simulink model "Flanging"  (R2018b)
settings: Solver=VariableStepAuto  StartTime=0.0  StopTime=10.0  RelTol=1e-3
libraries: dspsnks4 x1, dspvision x1
settings Model: Creator=alexa  LastModifiedBy=alexa

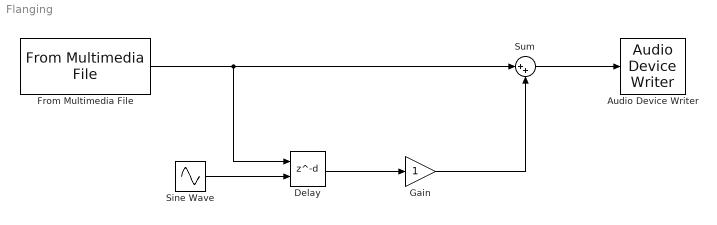
== system Flanging ==
  Audio Device Writer : dspsnks4/Audio Device Writer  Driver=DirectSound  Device=Default  InheritSampleRate=on  SampleRate=44100  BitDepth=16-bit integer  BufferSize=4096  NumBuffers=10  DefaultOutputChannelMapping=on  OutputChannelMapping=1:2  OutputNumUnderrunSamples=off  DriverIdx=1  DeviceWarnFlag=''
  Delay : Delay  DelayLengthSource=Input port
      settings: InputPortMap=u0,p1
  From Multimedia File : dspvision/From Multimedia File  inputFilename=C:\Users\alexa\OneDrive\Documents\Codigos PDS\Clase 3\Sonido.wav  loop=on  numPlays=inf  outputStreams=Audio only  videoDataType=single  audioDataType=double  inheritSampleTime=on  userDefinedSampleTime=1/30  noAudioOutput=off  isIntensityVideo=off  fourcc=RGB  colorVideoFormat=Separate color signals  outputEOF=off  dataOrg=Column-major  audioFrameSize=1024  computeAudioFrameSize=off  outSamplingMode=Sample based
      settings: SourceProductBaseCode=VP
  Gain : Gain
  Sine Wave : Sin  Amplitude=10  SampleTime=0
  Sum : Sum  Inputs=|++
  wires:
  From Multimedia File/1 -> Delay/1, Sum/1
  Sum/1 -> Audio Device Writer/1
  Gain/1 -> Sum/2
  Delay/1 -> Gain/1
  Sine Wave/1 -> Delay/2
